simulink model "A2"  (R2018a)
settings: Solver=VariableStepAuto  StartTime=0.0  StopTime=3  FixedStep=1  RelTol=1e-3
settings Model: Creator=U500304  LastModifiedBy=U500304

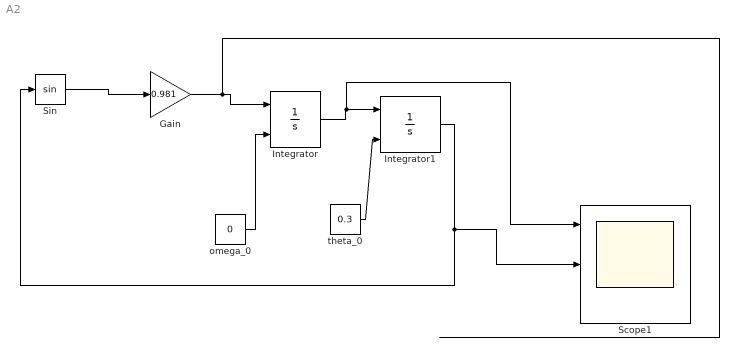
== system A2 ==
  Gain : Gain  Gain=0.981
  Integrator : Integrator  InitialConditionSource=external
  Integrator1 : Integrator  InitialConditionSource=external
  Scope1 : Scope  NumInputPorts=3
  Sin : Trigonometry
  "omega_0 " : Constant  Value=0  SampleTime=-1
  "theta_0 " : Constant  Value=0.3
  wires:
  "omega_0 "/1 -> Integrator/2
  "theta_0 "/1 -> Integrator1/2
  Integrator/1 -> Scope1/1, Integrator1/1
  Integrator1/1 -> Sin/1, Scope1/2
  Gain/1 -> Integrator/1
  Sin/1 -> Gain/1
